simulink model "Scope_trim_linmod"  (R2023b)
settings: Solver=VariableStepAuto  StartTime=0.0  StopTime=60  RelTol=1e-3
undefined symbols (not defined in the file or in its folder): A1, A21, A3, A4, A5, A6, A7, A8, B1, B2, B3, B4, B5, B6, B7, B8, C1, C2, C3, C4, C5, C6, C7, C8, D1, D2, D3, D4, D5, D6, D7, D8
settings Model: Creator=Stefaneko  LastModifiedBy=Stefaneko

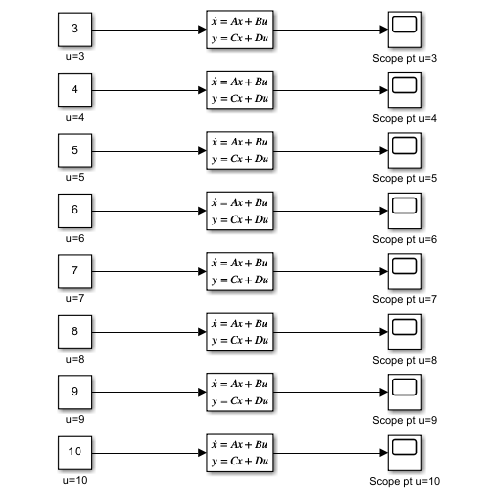
[thumbnail: Simulink's stored preview of the top-level diagram]
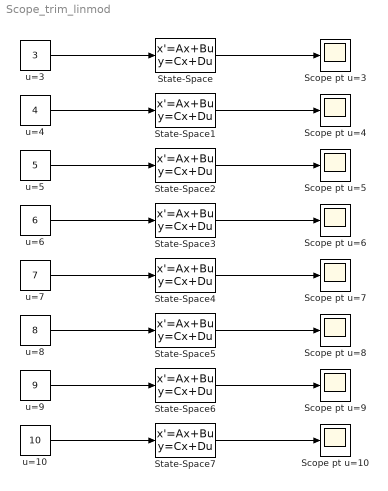
== system Scope_trim_linmod ==
  Scope pt u={3..10} (8 alike) : Scope
  State-Space : StateSpace  A=A1  B=B1  C=C1  D=D1  InitialCondition=0
  State-Space1 : StateSpace  A=A21  B=B2  C=C2  D=D2  InitialCondition=0
  State-Space2 : StateSpace  A=A3  B=B3  C=C3  D=D3  InitialCondition=0
  State-Space3 : StateSpace  A=A4  B=B4  C=C4  D=D4  InitialCondition=0
  State-Space4 : StateSpace  A=A5  B=B5  C=C5  D=D5  InitialCondition=0
  State-Space5 : StateSpace  A=A6  B=B6  C=C6  D=D6  InitialCondition=0
  State-Space6 : StateSpace  A=A7  B=B7  C=C7  D=D7  InitialCondition=0
  State-Space7 : StateSpace  A=A8  B=B8  C=C8  D=D8  InitialCondition=0
  u=10 : Constant  Value=10
  u=3 : Constant  Value=3
  u=4 : Constant  Value=4
  u=5 : Constant  Value=5
  u=6 : Constant  Value=6
  u=7 : Constant  Value=7
  u=8 : Constant  Value=8
  u=9 : Constant  Value=9
  wires:
  State-Space/1 -> Scope pt u=3/1
  u=3/1 -> State-Space/1
  State-Space1/1 -> Scope pt u=4/1
  u=4/1 -> State-Space1/1
  State-Space2/1 -> Scope pt u=5/1
  u=5/1 -> State-Space2/1
  State-Space3/1 -> Scope pt u=6/1
  u=6/1 -> State-Space3/1
  State-Space4/1 -> Scope pt u=7/1
  u=7/1 -> State-Space4/1
  State-Space5/1 -> Scope pt u=8/1
  u=8/1 -> State-Space5/1
  State-Space6/1 -> Scope pt u=9/1
  u=9/1 -> State-Space6/1
  State-Space7/1 -> Scope pt u=10/1
  u=10/1 -> State-Space7/1
